simulink model "Unbatch_Model"  (R2023a)
settings: Solver=VariableStepAuto  StartTime=0.0  StopTime=10.0  RelTol=1e-3
libraries: NSA_DEVS_LOGISTICS_ATOMIC x3, NSA_DEVS_SOURCES_ATOMIC x2, NSA_DEVS_SINKS_ATOMIC x1
settings Model: Creator=david  LastModifiedBy=david

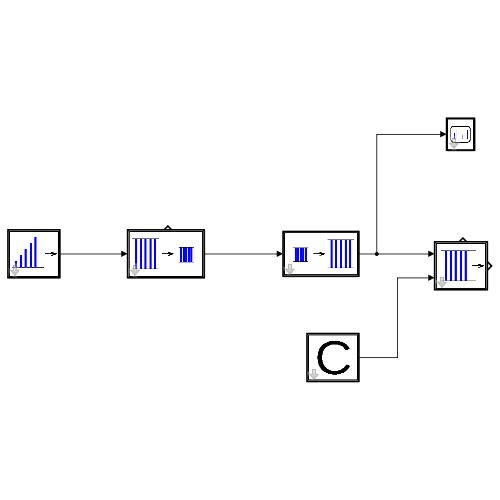
[thumbnail: Simulink's stored preview of the top-level diagram]
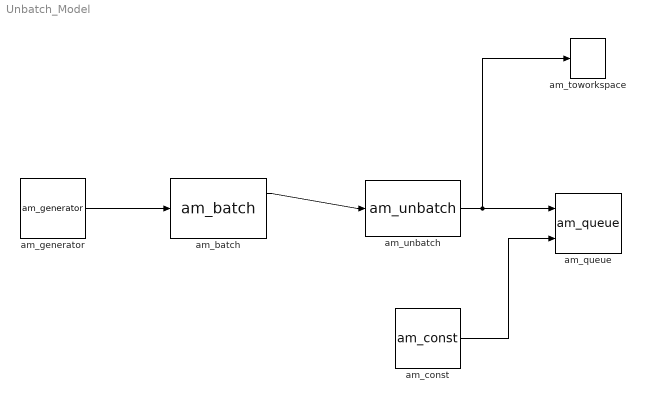
== system Unbatch_Model ==
  am_batch : NSA_DEVS_LOGISTICS_ATOMIC/am_batch  N=10  tau=[0,1]  debug=0
      settings: SourceProductName=NSA_DEVS
  am_const : NSA_DEVS_SOURCES_ATOMIC/am_const  value="\"1\""  sendTime=[0,1]  tau=[0,1]  debug=0
      settings: SourceProductName=NSA_DEVS
  am_generator : NSA_DEVS_SOURCES_ATOMIC/am_generator  tG=1  n0=0  nG=inf  tau=[0,1]  debug=0
      settings: SourceProductName=NSA_DEVS
  am_queue : NSA_DEVS_LOGISTICS_ATOMIC/am_queue  tD=[0,1]  tau=[0,1]  debug=0
      settings: SourceProductName=NSA_DEVS
  am_toworkspace : NSA_DEVS_SINKS_ATOMIC/am_toworkspace  varname="\"out\""  t0=0  format="\"vector\""  tau=[0,0.5]  debug=0
      settings: SourceProductName=NSA_DEVS
  am_unbatch : NSA_DEVS_LOGISTICS_ATOMIC/am_unbatch  tD=[0,1]  tau=[0,2]  debug=0
      settings: SourceProductName=NSA_DEVS
  wires:
  am_generator/1 -> am_batch/1
  am_batch/1 -> am_unbatch/1
  am_unbatch/1 -> am_toworkspace/1, am_queue/1
  am_const/1 -> am_queue/2
